simulink model "Controladro_por_bloques"  (R2022b)
settings: Solver=VariableStepAuto  StartTime=0.0  StopTime=10.0  RelTol=1e-3
InitFcn:
  | A = [1 2 0 -4; 0 1 2 -2; -3 -3 5 3;-2 2 4 4];
  | B = [0,0,0;0,0,0;-1,3,1;2,-6,3];
  | C = [-2 -2 0 0;0 1 0 0;1 2 2 0;-1 0 1 -1];
  | k1 = -4; k2 = -12;
settings Model: Creator=garci  LastModifiedBy=garci

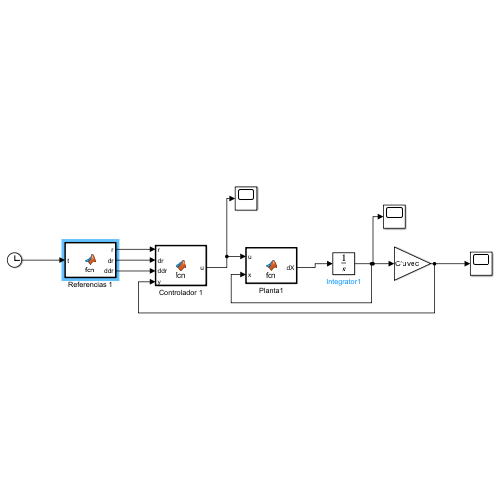
[thumbnail: Simulink's stored preview of the top-level diagram]
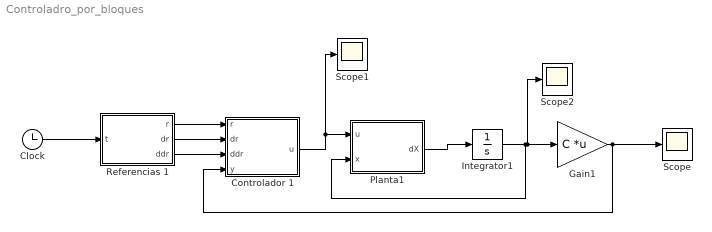
== system Controladro_por_bloques ==
  Clock : Clock
  Controlador 1 : MATLAB Function  TreatAsAtomicUnit=on
  Gain1 : Gain  Gain=C  Multiplication=Matrix(K*u) (u vector)
  Integrator1 : Integrator
  Planta1 : MATLAB Function  TreatAsAtomicUnit=on
  Referencias 1 : MATLAB Function  TreatAsAtomicUnit=on
  Scope : Scope
  Scope1 : Scope
  Scope2 : Scope
  wires:
  Clock/1 -> Referencias 1/1(t)
  Referencias 1/1(r) -> Controlador 1/1(r)
  Referencias 1/2(dr) -> Controlador 1/2(dr)
  Referencias 1/3(ddr) -> Controlador 1/3(ddr)
  Controlador 1/1(u) -> Scope1/1, Planta1/1(u)
  Planta1/1(dX) -> Integrator1/1
  Integrator1/1 -> Planta1/2(x), Scope2/1, Gain1/1
  Gain1/1 -> Controlador 1/4(y), Scope/1

== matlab function Controladro_por_bloques/Controlador 1 ==
  data: r input; u output; dr input; ddr input; y input; C parameter; A parameter; B parameter; k1 parameter; k2 parameter
function u = fcn(r,dr,ddr,y,C, A, B, k1, k2)

x = C^-1*y;
C12 = C(1:2,:);
%1er bloque 
e1 = r-y(1:2,:);
de1 = dr - C12*A*x;
x34R = [4 -12; -2 2]^-1 * (dr-[2 2;0 1]*x(1:2,:)-k1*e1);
%bloque 2
dx12 = A(1:2,:)*x;
dx34r = [4 -12;-2 2]^-1 * (ddr -[2 2;0 1]*dx12 - k1*de1);
e2 = x34R -x(3:4,:);
u = [0;B(3:4,2:3)^-1*(dx34r - A(3:4,:)*x - k2*e2)];

== matlab function Controladro_por_bloques/Planta1 ==
  data: u input; dX output; x input; A parameter; B parameter
function dX = fcn(u, x, A, B)

dX = A*x + B*u;

== matlab function Controladro_por_bloques/Referencias 1 ==
  data: t input; r output; dr output; ddr output
function [r, dr, ddr] = fcn(t)

r = [7;5];
dr = [0;0];
ddr = [0;0];
